simulink model "ACCMPC"  (R2023b)
settings: Solver=FixedStepDiscrete  StartTime=0.0  StopTime=1800  FixedStep=0.005  MaxStep=0.005  RelTol=1e-3  EnableMultiTasking=on
InitFcn:
  | load('DrivingCycles/WLTC.mat')
  | load('DrivingCycles/Mappa_Throttle.mat')
model workspace: external: MATLAB File C:\Users\stefa\Documents\EEPACC_MPC_CasADi_MATLAB\ACCMPC-ABO_CasADi\Init_ACCMPC_sim.m (data not in the file)
values from neighbouring files (symbols this model uses):
  OPTsettings = Settings(OPTsettings)    [Init_ACCMPC_sim.m]    (also in Main.m; Settings.m = GenerateUseCase(OPTsettings))
  V = SetVehicleParameters()    [Custom_plots.m]    (also in Init_ACCMPC_sfun.m; Init_ACCMPC_sim.m; Main.m; RunInit_ABMPC_sfun.m = SetParametersInternally())
undefined symbols (not defined in the file or in its folder): DiscIntNeverNeededParam, throttle_pedal, wheel_speed_radps, wheel_torque_Nm
libraries: slpidlib x4, simulink x1
(part 2 of 2)

== matlab function ACCMPC/Low Level Controller and Plant/MATLAB Function ==
  data: v input; power_w output; dvdt input; RG input
function power_w   = vehFcn(v, dvdt, RG)
%vehFcn  ODE file representing the dynamics of the longitudinal speed.

% use: [t,v] = ode45(@(t,v) vehFcn(t, v, u, theta), tspan, v0);  % One comma removed
persistent m Tm wm Beta a_n gear  g 
 if isempty(m)
     m       = 3283;     % kg mass
     g       = 9.8;      % m/s2
     Tm      = 390;      % Nm
     wm      = 418.8790; % rad/s (about 4000 RPM),;      % rad/s (about 4000 RPM),
     Beta    = 0.4;      % 
     %r      = 0.6;      % m - loaded wheel radious
     a_n     = [47.2 33.2 21.1 16.7 12.9 10.0 8.4 6.7]'; 

     % variables updated internaly:
     gear    = 1;

 end

theta = atan(RG/100);
%% intermediate eqs:
% gear selection:
if v <= 6  
   gear = 1;  
elseif v > 6 && v <= 10 
   gear = 2;
elseif v > 10 && v <= 13
   gear = 3;
elseif v > 13 && v <= 18
   gear = 4;
elseif v > 18 && v <= 24
   gear = 5;
elseif v > 24 && v <= 33
   gear = 6;
elseif v > 33 && v <= 41
   gear = 7;  
elseif v > 41
   gear = 8;  
end

% engine speed:
w = a_n(gear)*v;
% w = n/r*v

% engine torque:
Te = Tm*(1 - Beta*(w/wm-1)^2);

F0 = 345;
F1 = 0;
F2 = 0.1007/(1/3.6)^2;

% gravity force:
Fg = m*g*sin(theta);

% State equations.
Ftotal = max(m*dvdt + (F0 + F1*v + F2*v^2 + Fg), 0);
power_w = Ftotal*v;

== matlab function ACCMPC/Scenario - RADAR/MATLAB Function ==
  data: v input; power_w output; dvdt input; RG input
function power_w   = vehFcn(v, dvdt, RG)
%vehFcn  ODE file representing the dynamics of the longitudinal speed.

% use: [t,v] = ode45(@(t,v) vehFcn(t, v, u, theta), tspan, v0);  % One comma removed
persistent m Tm wm Beta a_n gear  g 
 if isempty(m)
     m       = 3283;     % kg mass
     g       = 9.8;      % m/s2
     Tm      = 390;      % Nm
     wm      = 418.8790; % rad/s (about 4000 RPM),;      % rad/s (about 4000 RPM),
     Beta    = 0.4;      % 
     %r      = 0.6;      % m - loaded wheel radious
     a_n     = [47.2 33.2 21.1 16.7 12.9 10.0 8.4 6.7]'; 

     % variables updated internaly:
     gear    = 1;

 end

theta = atan(RG/100);
%% intermediate eqs:
% gear selection:
if v <= 6  
   gear = 1;  
elseif v > 6 && v <= 10 
   gear = 2;
elseif v > 10 && v <= 13
   gear = 3;
elseif v > 13 && v <= 18
   gear = 4;
elseif v > 18 && v <= 24
   gear = 5;
elseif v > 24 && v <= 33
   gear = 6;
elseif v > 33 && v <= 41
   gear = 7;  
elseif v > 41
   gear = 8;  
end

% engine speed:
w = a_n(gear)*v;
% w = n/r*v

% engine torque:
Te = Tm*(1 - Beta*(w/wm-1)^2);

F0 = 345;
F1 = 0;
F2 = 0.1007/(1/3.6)^2;

% gravity force:
Fg = m*g*sin(theta);

% State equations.
Ftotal = max(m*dvdt + (F0 + F1*v + F2*v^2 + Fg), 0) ; 
power_w = Ftotal*v;

== matlab function ACCMPC/Plant Model ==
  data: x_0 input; u input; OPTsettings input; s_measured output size=1; v_measured output
function [s_measured, v_measured] = RunPlantModel(x_0,u,OPTsettings)
% RunPlantModel Nonlinear model to simulate the real plant and get the next state with a given control input. 
% The model uses RK4 with a set number of steps for integration.
%
%   Inputs:
%       x_0         : initial state  := [s_0,v_0]
%       u           : control signal := [F_m,F_b]
%       OPTsettings : struct with settings for the MPC
%
%   Outputs:
%       s_measured : simulated measured travel distance in the next step
%       v_measured : simulated measured velocity in the next step

    %% Initialization

    s_slope = OPTsettings.s_slope;          % PWA slope function distances
    slope   = OPTsettings.slope;            % PWA slope function values
    M       = OPTsettings.N_integratePlant; % number of RK4 steps
    Ts      = OPTsettings.Tvec(1);          % sample time of the controller
    V       = SetVehicleParameters();       % vehicle parameters
    u_k     = sum(u);                       % total force
    DT      = Ts/M;                         % time step per interval
    x_k     = x_0;                          % initial state

    %% Fixed step Runge-Kutta 4 integration
    
    % Run M RK4 integration steps
    for k=1:M
        k1 = f_NL(x_k          , u_k, s_slope, slope);
        k2 = f_NL(x_k + DT/2*k1, u_k, s_slope, slope);
        k3 = f_NL(x_k + DT/2*k2, u_k, s_slope, slope);
        k4 = f_NL(x_k + DT  *k3, u_k, s_slope, slope);
        x_k = x_k + DT/6*(k1 + 2*k2 + 2*k3 + k4);
    end

    % set the measurement simulation result
    s_measured = x_k(1);
    v_measured = x_k(2);
    
    %% Function containing the nonlinear dynamics

    function x_dot = f_NL(x_k, u_k, s_slope, slope)
        theta = InterpPWA(x_k(1),s_slope,slope);
        x_dot = [x_k(2), 1/V.lambda/V.m*(u_k - V.zeta_a*x_k(2)^2 - V.c_r*V.m*V.g*cos(theta) - V.m*V.g*sin(theta))];
    end

end

== matlab function ACCMPC/ACC /Estimate EGO Vehicle Trajectory ==
  data: OPTsettings input; estSetting input; s_curr input; s_est output size=1; v_est output; v_curr input; a_curr input; s_opt_prev_sol input; v_opt_prev_sol input
function [s_est, v_est] = EstimateVehicleTrajectory(OPTsettings, estSetting, s_curr, v_curr, a_curr, s_opt_prev_sol, v_opt_prev_sol)
% EstimateVehicleTrajectory Estimates the trajectory of the target or ego vehicle along the prediction horizon
%
%   Inputs:
%       OPTsettings    : struct with settings for the optimization
%       estSetting     : (0) estimate ego vehicle trajectory for FBMPC or ABMPC; (1) estimate target vehicle trajectory; (2) estimation for the TVMPC; (3) estimation for the BLMPC
%       s_curr         : current travel distance for the estimate
%       v_curr         : current velocity for the estimate
%       a_curr         : current acceleration for the estimate
%       s_opt_prev_sol : optimal solution for the travel distance in the horizon of the previous QP
%       v_opt_prev_sol : optimal solution for the velocity in the horizon of the previous QP
%
%   Outputs:
%       s_est          : estimate of the travel distance along the horizon
%       v_est          : estimate of the velocity along the horizon
        
    %% initialization

    % extract settings
    if estSetting == 2
        % for TVMPC
        paramEstSetting = OPTsettings.TV_trajEstSett;
        Ts              = OPTsettings.TV_Ts;
        N_hor           = OPTsettings.TV_N_hor;
    elseif estSetting == 3
        % for BLMPC
        paramEstSetting = OPTsettings.BL_trajEstSett;
        Ts              = OPTsettings.BL_Ts;
        N_hor           = OPTsettings.BL_N_hor;
    else
        % for ABMPC and FBPMC
        N_hor = OPTsettings.N_hor;
        Tvec  = OPTsettings.Tvec;
        if estSetting == 0
            paramEstSetting = OPTsettings.paramEstSetting;
        else
            paramEstSetting = OPTsettings.TVestSetting;
        end
    end

    % const. acceleration time when using paramEstSetting 2
    if estSetting == 1
        tConstACC = OPTsettings.tConstACC_tar;
    else
        tConstACC = OPTsettings.tConstACC_ego;
    end

    % initialize arrays
    s_est = zeros(N_hor+1,1);
    v_est = zeros(N_hor+1,1);

    %% Estimation

    % Estimate distance and velocity for the full horizon
    if paramEstSetting == 0
        % constant velocity
        s_est(1) = s_curr;
        for i = 2:N_hor+1
            if estSetting < 2
                Ts = Tvec(i-1);
            end
            s_est(i) = s_est(i-1) + Ts*v_curr;
        end
        v_est = v_curr*ones(1,N_hor+1);
    elseif paramEstSetting == 1
        % constant acceleration
        s_est(1) = s_curr;
        v_est(1) = v_curr;
        for i = 2:N_hor+1
            if estSetting < 2
                Ts = Tvec(i-1);
            end
            if i <= tConstACC/Ts && v_est(i-1) + Ts*a_curr > 0
                v_est(i) = v_est(i-1) + Ts*a_curr;
            else
                v_est(i) = v_est(i-1);
            end
            s_est(i) = s_est(i-1) + Ts*v_est(i-1);
            
        end
    else
        if estSetting < 2
            Ts = Tvec(end);
        end
        % use the previous MPC solutions
        s_est = [s_curr; s_opt_prev_sol(3:end); s_opt_prev_sol(end)+Ts*v_opt_prev_sol(end)];
        v_est = [v_curr; v_opt_prev_sol(3:end); v_opt_prev_sol(end)];
    end

end
